simulink model "Copy_of_Lab2_single_loop_controller_student"  (R2024b)
settings: Solver=ode45  StartTime=0.0  StopTime=10  MaxStep=0.01  RelTol=1e-3
values from neighbouring files (symbols this model uses):
  kt = 5.06e-2    (= 0.0506)    [Lab2_params_student.m]    (also in cascade_araigordai.mat)
  Lm = 2.84e-3    (= 0.00284)    [Lab2_params_student.m]    (also in cascade_araigordai.mat)
  R = 3.18    [Lab2_params_student.m]    (also in cascade_araigordai.mat)
  time = kp_1{2}.Values.Time    [FindRequirementValues.m]    (also in Lab2_params_student.m = 0.000893081761006; absloute_tracking_error.m = cascade_try{2}.Values.Time; cascade_araigordai.mat = [0 5.09224491077e-30 0.000393993366556 0.000714758903211 0.0; state1.m = cascade_try{2}.Values.Time)
settings Model: Creator=User  LastModifiedBy=bpbeam
settings RTWCC: GPUComputeCapability=3.5

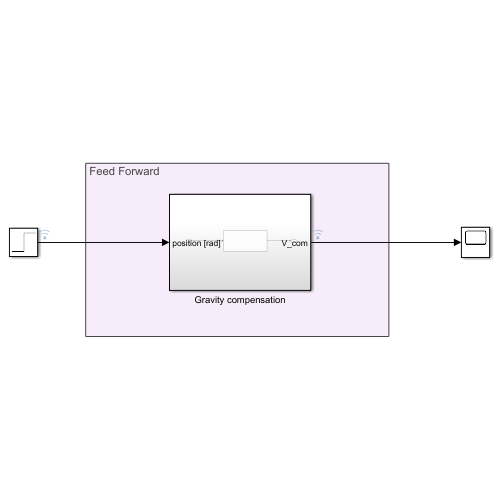
[thumbnail: Simulink's stored preview of the top-level diagram]
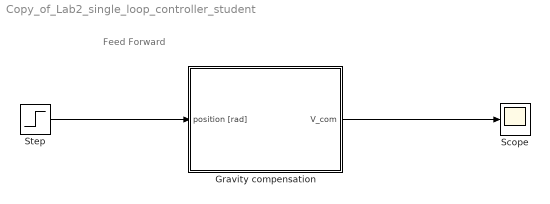
== system Copy_of_Lab2_single_loop_controller_student ==
  note: Feed Forward
  Gravity compensation : Subsystem
  Scope : Scope
  Step : Step  SampleTime=0
  wires:
  Step/1 -> Gravity compensation/1(position [rad])
  Gravity compensation/1(V_com) -> Scope/1

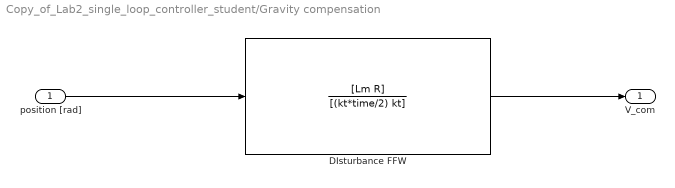
== system Copy_of_Lab2_single_loop_controller_student/Gravity compensation ==
  position [rad] : Inport
  DIsturbance FFW : TransferFcn  Numerator=[Lm R]  Denominator=[(kt*time/2) kt]
  V_com : Outport
  wires:
  position [rad]/1 -> DIsturbance FFW/1
  DIsturbance FFW/1 -> V_com/1
